simulink library "relFlowCoeff2qua"  (R2018b)
settings: Solver=ode45  StartTime=0.0  StopTime=10.0  RelTol=1e-3  EnableMultiTasking=on
libraries: carnot x1
settings Model: Creator=lena.frank  LastModifiedBy=P41573
settings DataIOCC: LimitDataPoints=on  SaveFormat=Array  SignalLoggingSaveFormat=ModelDataLogs
settings OptimizationCC: ExpressionDepthLimit=2147483647  LifeSpan=inf
settings DebuggingCC: UnderspecifiedInitializationDetection=Classic  MergeDetectMultiDrivingBlocksExec=none  SolverPrmCheckMsg=warning  FcnCallInpInsideContextMsg=warning  StateNameClashWarn=warning  SFUnexpectedBacktrackingDiag=warning  SFNoUnconditionalDefaultTransitionDiag=warning  SFExecutionAtInitializationDiag=none
settings HardwareCC: ProdBitPerPointer=32  ProdBitPerSizeT=32  ProdBitPerPtrDiffT=32  ProdLargestAtomicFloat=None  ProdIntDivRoundTo=Undefined  ProdEndianess=Unspecified  ProdWordSize=32  ProdHWDeviceType=32-bit Generic
settings ModelReferenceCC: PropagateSignalLabelsOutOfModel=off
settings SFSimCC: SimUseLocalCustomCode=off
settings RTWCC: RTWUseLocalCustomCode=off
settings CodeAppCC: StateflowObjectComments=on
settings GRTTargetCC: TargetLangStandard=C89/C90 (ANSI)  GeneratePreprocessorConditionals=Disable all  CombineOutputUpdateFcns=off  GRTInterface=on
settings ConfigComp: CovMetricSettings=dw  CovHtmlReporting=on  CovSaveCumulativeToWorkspaceVar=on  CovSaveSingleToWorkspaceVar=on  CovExternalEMLEnable=off

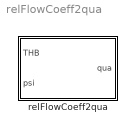
== system relFlowCoeff2qua ==
  relFlowCoeff2qua : Subsystem  mask{kvs=1.6}
      mask prompts: kvs "Flow coefficient of open valve (Kvs) in m³/h"
      mask TypeOptions kvs: Kvs/Gain
      mask Display: disp('rel\nFlow Coeff\nto qua')

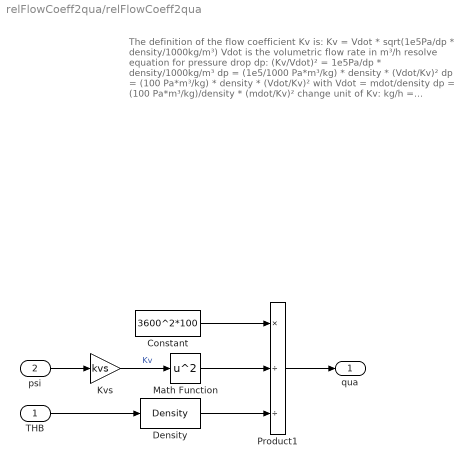
== system relFlowCoeff2qua/relFlowCoeff2qua ==
  note: The definition of the flow coefficient Kv is:
      | Kv = Vdot * sqrt(1e5Pa/dp * density/1000kg/m³)
      | Vdot is the volumetric flow rate in m³/h
      | resolve equation for pressure drop dp:
      | (Kv/Vdot)² = 1e5Pa/dp * density/1000kg/m³
      | dp = (1e5/1000 Pa*m³/kg) * density * (Vdot/Kv)²
      | dp = (100 Pa*m³/kg) * density * (Vdot/Kv)²
      | with Vdot = mdot/density
      | dp = (100 Pa*m³/kg)/density * (mdot/Kv)²
      | change unit of Kv: kg/h = kg/(3600s)
      | dp = (100 Pa*m³/kg) * (3600 s/h)² / density * (mdot/Kv)²
      | Carnot equation: dp = qua * mdot²
      | qua = (100 Pa*m³/kg) * (3600 s/h)² / (density*Kv²)
  THB : Inport
  psi : Inport  Port=2
  Constant : Constant  Value=3600^2*100
  Density : carnot/Basic/Material_Properties/Density  VariantControl=CarlibClassic  INPUTARGUMENTS=THB  DEBUGLEVEL=DEBUGLEVEL  MAXTOTALWARNINGS=inf  MAXCONSECUTIVEWARNINGS=inf  WRITETOFILE=0  FILENAME='errors.txt'
      settings: SourceProductName=Carnot
  Kvs : Gain  Gain=kvs
  Math Function : Math  Operator=square  SaturateOnIntegerOverflow=on
  Product1 : Product  Inputs=*//
  qua : Outport
  wires:
  Kvs/1 -> Math Function/1  "Kv"
  psi/1 -> Kvs/1
  Constant/1 -> Product1/1
  Product1/1 -> qua/1
  Math Function/1 -> Product1/2
  Density/1 -> Product1/3
  THB/1 -> Density/1
